simulink model "Scenario_3_v2"  (R2020b)
settings: Solver=ode1be  StartTime=0.0  StopTime=0.5  FixedStep=Ts  MaxStep=Ts/10  MinStep=Ts/40  RelTol=1e-3
values from neighbouring files (symbols this model uses):
  c0 = c0_zeb    (= 6.57988e-09)    [Scenario_17_parameters_v2.m]    (also in Scenario_1_parameters_v2.m; Scenario_2_parameters_v2.m; Scenario_3_parameters_v2.m)
  c0_hawk = 6.37282e-09    [Scenario_17_parameters_v2.m]    (also in Scenario_1_parameters_v2.m; Scenario_2_parameters_v2.m; Scenario_3_parameters_v2.m)
  c1 = c1_zeb    (= 9.15905e-09)    [Scenario_17_parameters_v2.m]    (also in Scenario_1_parameters_v2.m; Scenario_2_parameters_v2.m; Scenario_3_parameters_v2.m)
  c1_hawk = 8.76156e-09    [Scenario_17_parameters_v2.m]    (also in Scenario_1_parameters_v2.m; Scenario_2_parameters_v2.m; Scenario_3_parameters_v2.m)
  fg = 50    [Scenario_17_parameters_v2.m]    (also in Scenario_1_parameters_v2.m; Scenario_2_parameters_v2.m; Scenario_3_parameters_v2.m)
  G10gen = 0.90    (= 0.9)    [Scenario_3_parameters_v2.m]
  G12gen = 0.85    [Scenario_3_parameters_v2.m]
  G1gen = 0.4692    [Scenario_17_parameters_v2.m]    (also in Scenario_1_parameters_v2.m = 0.1; Scenario_2_parameters_v2.m = 0.298581; Scenario_3_parameters_v2.m = 0.65)
  G2gen = 0.80    (= 0.8)    [Scenario_1_parameters_v2.m]    (also in Scenario_2_parameters_v2.m = 0.7; Scenario_3_parameters_v2.m = 0.4)
  G3gen = 0.85    [Scenario_1_parameters_v2.m]    (also in Scenario_2_parameters_v2.m = 0.9; Scenario_3_parameters_v2.m = 0.6)
  G4gen = 0.65    [Scenario_3_parameters_v2.m]
  G5gen = 0.75    [Scenario_17_parameters_v2.m]    (also in Scenario_1_parameters_v2.m = 0.8; Scenario_2_parameters_v2.m = 0.8; Scenario_3_parameters_v2.m = 0.705)
  G6gen = 0.90    (= 0.9)    [Scenario_17_parameters_v2.m]    (also in Scenario_1_parameters_v2.m; Scenario_2_parameters_v2.m = 0.81797; Scenario_3_parameters_v2.m = 0.45)
  G7gen = 0.20    (= 0.2)    [Scenario_17_parameters_v2.m]    (also in Scenario_1_parameters_v2.m = 0.5227; Scenario_2_parameters_v2.m = 0.5098; Scenario_3_parameters_v2.m = 0.4)
  G8gen = 0.58    [Scenario_17_parameters_v2.m]    (also in Scenario_3_parameters_v2.m = 0.65)
  G9gen = 0.8833    [Scenario_17_parameters_v2.m]    (also in Scenario_3_parameters_v2.m = 0.9)
  Iovc = 1.2    [Scenario_17_parameters_v2.m]    (also in Scenario_1_parameters_v2.m; Scenario_2_parameters_v2.m; Scenario_3_parameters_v2.m)
  l0 = l0_zeb    (= 0.00368)    [Scenario_17_parameters_v2.m]    (also in Scenario_1_parameters_v2.m; Scenario_2_parameters_v2.m; Scenario_3_parameters_v2.m)
  l0_hawk = 0.00373    [Scenario_17_parameters_v2.m]    (also in Scenario_1_parameters_v2.m; Scenario_2_parameters_v2.m; Scenario_3_parameters_v2.m)
  l1 = l1_zeb    (= 0.00128)    [Scenario_17_parameters_v2.m]    (also in Scenario_1_parameters_v2.m; Scenario_2_parameters_v2.m; Scenario_3_parameters_v2.m)
  L10dem = 0.04    [Scenario_3_parameters_v2.m]
  L12dem = 0.01    [Scenario_17_parameters_v2.m]    (also in Scenario_3_parameters_v2.m = 0.02)
  L13dem = 0.01    [Scenario_3_parameters_v2.m]
  l1_hawk = 0.00133    [Scenario_17_parameters_v2.m]    (also in Scenario_1_parameters_v2.m; Scenario_2_parameters_v2.m; Scenario_3_parameters_v2.m)
  L1dem = 0.25    [Scenario_17_parameters_v2.m]    (also in Scenario_3_parameters_v2.m = 0.1)
  L3dem = 0.30    (= 0.3)    [Scenario_17_parameters_v2.m]    (also in Scenario_1_parameters_v2.m = 0.1; Scenario_2_parameters_v2.m = 0.1; Scenario_3_parameters_v2.m = 0.2)
  L5dem = 0.25    [Scenario_17_parameters_v2.m]    (also in Scenario_1_parameters_v2.m = 0.35; Scenario_2_parameters_v2.m = 0.35; Scenario_3_parameters_v2.m = 0.1)
  L6dem = 0.15    [Scenario_1_parameters_v2.m]    (also in Scenario_2_parameters_v2.m; Scenario_3_parameters_v2.m = 0.1)
  L7dem = 0.10    (= 0.1)    [Scenario_1_parameters_v2.m]    (also in Scenario_2_parameters_v2.m; Scenario_3_parameters_v2.m = 0.2)
  L9dem = 0.15    [Scenario_17_parameters_v2.m]    (also in Scenario_3_parameters_v2.m = 0.1)
  Pr = Sr*PF    (= 1600500000)    [Scenario_17_parameters_v2.m]    (also in Scenario_1_parameters_v2.m = 1472500000; Scenario_2_parameters_v2.m = 1805000000; Scenario_3_parameters_v2.m = 12740000000)
  Qr = sqrt(Sr^2 - Pr^2)    [Scenario_17_parameters_v2.m]    (also in Scenario_1_parameters_v2.m; Scenario_2_parameters_v2.m; Scenario_3_parameters_v2.m)
  r0 = r0_zeb    (= 0.39362)    [Scenario_17_parameters_v2.m]    (also in Scenario_1_parameters_v2.m; Scenario_2_parameters_v2.m; Scenario_3_parameters_v2.m)
  r0_hawk = 0.44587    [Scenario_17_parameters_v2.m]    (also in Scenario_1_parameters_v2.m; Scenario_2_parameters_v2.m; Scenario_3_parameters_v2.m)
  r1 = r1_zeb    (= 0.06862)    [Scenario_17_parameters_v2.m]    (also in Scenario_1_parameters_v2.m; Scenario_2_parameters_v2.m; Scenario_3_parameters_v2.m)
  r1_hawk = 0.12087    [Scenario_17_parameters_v2.m]    (also in Scenario_1_parameters_v2.m; Scenario_2_parameters_v2.m; Scenario_3_parameters_v2.m)
  Rtpu = Xtpu/40    (= 0.0025)    [Scenario_17_parameters_v2.m]    (also in Scenario_1_parameters_v2.m = 0.00375; Scenario_2_parameters_v2.m = 0.00375; Scenario_3_parameters_v2.m)
  S10non = 500e6    (= 500000000)    [Scenario_3_parameters_v2.m]
  S12non = 250e6    (= 250000000)    [Scenario_3_parameters_v2.m]
  S1non = 700e6    (= 700000000)    [Scenario_17_parameters_v2.m]    (also in Scenario_1_parameters_v2.m = 400000000; Scenario_2_parameters_v2.m = 400000000; Scenario_3_parameters_v2.m = 1000000000)
  S2non = 300e6    (= 300000000)    [Scenario_1_parameters_v2.m]    (also in Scenario_2_parameters_v2.m; Scenario_3_parameters_v2.m = 3000000000)
  S3non = 200e6    (= 200000000)    [Scenario_1_parameters_v2.m]    (also in Scenario_2_parameters_v2.m; Scenario_3_parameters_v2.m = 1000000000)
  S4non = 2000e6    (= 2000000000)    [Scenario_3_parameters_v2.m]
  S5non = 400e6    (= 400000000)    [Scenario_17_parameters_v2.m]    (also in Scenario_1_parameters_v2.m = 500000000; Scenario_2_parameters_v2.m = 500000000; Scenario_3_parameters_v2.m = 2000000000)
  S6non = 150e6    (= 150000000)    [Scenario_17_parameters_v2.m]    (also in Scenario_1_parameters_v2.m = 400000000; Scenario_2_parameters_v2.m = 400000000; Scenario_3_parameters_v2.m = 3000000000)
  S7non = 1500e6    (= 1500000000)    [Scenario_17_parameters_v2.m]    (also in Scenario_1_parameters_v2.m = 200000000; Scenario_2_parameters_v2.m = 200000000; Scenario_3_parameters_v2.m = 4000000000)
  S8non = 600e6    (= 600000000)    [Scenario_17_parameters_v2.m]    (also in Scenario_3_parameters_v2.m = 2000000000)
  S9non = 200e6    (= 200000000)    [Scenario_17_parameters_v2.m]    (also in Scenario_3_parameters_v2.m = 1500000000)
  tonvsc = 0    [Scenario_17_parameters_v2.m]    (also in Scenario_1_parameters_v2.m; Scenario_2_parameters_v2.m; Scenario_3_parameters_v2.m = 0.0001)
  Ts = 50e-6    (= 5e-05)    [Scenario_17_parameters_v2.m]    (also in Scenario_1_parameters_v2.m = 0.0002; Scenario_2_parameters_v2.m = 2e-05; Scenario_3_parameters_v2.m = 0.0001)
  Vhv = 220e3    (= 220000)    [Scenario_17_parameters_v2.m]    (also in Scenario_1_parameters_v2.m; Scenario_2_parameters_v2.m; Scenario_3_parameters_v2.m)
  Vmv = 22e3    (= 22000)    [Scenario_17_parameters_v2.m]    (also in Scenario_1_parameters_v2.m; Scenario_2_parameters_v2.m; Scenario_3_parameters_v2.m)
  w_pll = 2*pi*80    (= 502.654824574)    [Scenario_17_parameters_v2.m]    (also in Scenario_1_parameters_v2.m; Scenario_2_parameters_v2.m; Scenario_3_parameters_v2.m)
  wc1 = wsw1/10    (= 848.230016469)    [Scenario_17_parameters_v2.m]    (also in Scenario_1_parameters_v2.m; Scenario_2_parameters_v2.m; Scenario_3_parameters_v2.m)
  wdc1 = wc1/10    (= 84.8230016469)    [Scenario_17_parameters_v2.m]    (also in Scenario_1_parameters_v2.m; Scenario_2_parameters_v2.m; Scenario_3_parameters_v2.m)
  wpq1 = wc1/10    (= 84.8230016469)    [Scenario_17_parameters_v2.m]    (also in Scenario_1_parameters_v2.m; Scenario_2_parameters_v2.m; Scenario_3_parameters_v2.m)
  wsw1 = ksw1*2*pi*fg    (= 8482.30016469)    [Scenario_17_parameters_v2.m]    (also in Scenario_1_parameters_v2.m; Scenario_2_parameters_v2.m; Scenario_3_parameters_v2.m)
  Xtpu = 0.10    (= 0.1)    [Scenario_17_parameters_v2.m]    (also in Scenario_1_parameters_v2.m = 0.15; Scenario_2_parameters_v2.m = 0.15; Scenario_3_parameters_v2.m)
undefined symbols (not defined in the file or in its folder): D11, Delta
libraries: powerlib x428, simulink_extras x272, powerlib_meascontrol x194, pid_lib x105, simulink x60, eeTransforms x54, spsFirstOrderFilterLib x36, eePwmGeneratorTwoLevel x9
(part 10 of 40)

== system Scenario_3_v2/G7/VSC v2/VSC Model ==
  Ref : Inport
  EMT AVG : Subsystem  VariantControl=EMT_AVG
      settings: PortSchema="{\"entries\":[{\"content\":{\"sides\":[{\"content\":{\"connectorIds\":[\"LConn1\",\"LConn2\",\"LConn3\"]},\"type\":\"ConnectorPlacement.EquallySpacedRectSide\",\"uuid\":\"96043b84-a665-4cb2-a938-d6633d7ee474\"},{\"content\":{\"connectorIds\":[\"In1\"],\"side\":\"RIGHT\"},\"type\":\"ConnectorPlacement.EquallySpacedRectSide\",\"uuid\":\"064d463f-c23a-42ac-89ce-8dea3d446214\"},{\"content\":{\"connectorIds\":[],\"side\":\"TOP\"},\"type\":\"ConnectorPlacement.EquallySpacedRectSide\",\"uuid\":\"95ef669c-c6ed-44c3-8b69-447906728b6d\"}]},\"type\":\"ConnectorPlacement.EquallySpacedConnector\",\"uuid\":\"ea66db09-64d7-4d7e-ba7b-d769c56e2dbd\"}],\"packageUris\":[\"http://schema.mathworks.com/mf0/Connector/19700101\"],\"version\":\"1.0\"}"
  EMT SW : Subsystem  VariantControl=EMT_SW
      settings: PortSchema="{\"entries\":[{\"content\":{\"sides\":[{\"content\":{\"connectorIds\":[\"LConn1\",\"LConn2\",\"LConn3\"]},\"type\":\"ConnectorPlacement.EquallySpacedRectSide\",\"uuid\":\"96043b84-a665-4cb2-a938-d6633d7ee474\"},{\"content\":{\"connectorIds\":[\"In1\"],\"side\":\"RIGHT\"},\"type\":\"ConnectorPlacement.EquallySpacedRectSide\",\"uuid\":\"064d463f-c23a-42ac-89ce-8dea3d446214\"},{\"content\":{\"connectorIds\":[],\"side\":\"TOP\"},\"type\":\"ConnectorPlacement.EquallySpacedRectSide\",\"uuid\":\"95ef669c-c6ed-44c3-8b69-447906728b6d\"}]},\"type\":\"ConnectorPlacement.EquallySpacedConnector\",\"uuid\":\"ea66db09-64d7-4d7e-ba7b-d769c56e2dbd\"}],\"packageUris\":[\"http://schema.mathworks.com/mf0/Connector/19700101\"],\"version\":\"1.0\"}"
  Phasor : Subsystem  VariantControl=Phasor
      settings: PortSchema="{\"entries\":[{\"content\":{\"sides\":[{\"content\":{\"connectorIds\":[\"LConn1\",\"LConn2\",\"LConn3\"]},\"type\":\"ConnectorPlacement.EquallySpacedRectSide\",\"uuid\":\"96043b84-a665-4cb2-a938-d6633d7ee474\"},{\"content\":{\"connectorIds\":[\"In1\"],\"side\":\"RIGHT\"},\"type\":\"ConnectorPlacement.EquallySpacedRectSide\",\"uuid\":\"064d463f-c23a-42ac-89ce-8dea3d446214\"},{\"content\":{\"connectorIds\":[],\"side\":\"TOP\"},\"type\":\"ConnectorPlacement.EquallySpacedRectSide\",\"uuid\":\"95ef669c-c6ed-44c3-8b69-447906728b6d\"}]},\"type\":\"ConnectorPlacement.EquallySpacedConnector\",\"uuid\":\"ea66db09-64d7-4d7e-ba7b-d769c56e2dbd\"}],\"packageUris\":[\"http://schema.mathworks.com/mf0/Connector/19700101\"],\"version\":\"1.0\"}"
  A : PMIOPort  Side=Left
  B : PMIOPort  Port=2  Side=Left
  C : PMIOPort  Port=3  Side=Left

== system Scenario_3_v2/G7/VSC v2/output signals ==
  Vs : Inport
  Is : Inport  Port=2
  control : Inport  Port=3
  Bus Creator : BusCreator  Inputs=15
  Demux : Demux  Outputs=13
  m : Outport
  wires:
  Bus Creator/1 -> m/1
  control/1 -> Demux/1
  Vs/1 -> Bus Creator/1  "Vabc"
  Is/1 -> Bus Creator/2  "Iabc"
  Demux/1 -> Bus Creator/3  "vqp"
  Demux/2 -> Bus Creator/4  "vdp"
  Demux/3 -> Bus Creator/5  "vqn"
  Demux/4 -> Bus Creator/6  "vdn"
  Demux/5 -> Bus Creator/7  "iqp"
  Demux/6 -> Bus Creator/8  "idp"
  Demux/7 -> Bus Creator/9  "iqn"
  Demux/8 -> Bus Creator/10  "idn"
  Demux/9 -> Bus Creator/11  "f"
  Demux/10 -> Bus Creator/12  "Pdq"
  Demux/11 -> Bus Creator/13  "Qdq"
  Demux/12 -> Bus Creator/14  "Pabc"
  Demux/13 -> Bus Creator/15  "Qabc"

== system Scenario_3_v2/G9/VSC v2/VI measurement ==
  Current Measurement : powerlib/Measurements/Current Measurement  PhasorSimulation=off  OutputType=Complex  PSBequivalent=0
  Current Measurement1 : powerlib/Measurements/Current Measurement  PhasorSimulation=off  OutputType=Complex  PSBequivalent=0
  Current Measurement2 : powerlib/Measurements/Current Measurement  PhasorSimulation=off  OutputType=Complex  PSBequivalent=0
  Ground : powerlib/Elements/Ground  LConnTagsString=a
  Ground1 : powerlib/Elements/Ground  LConnTagsString=a
  Ground2 : powerlib/Elements/Ground  LConnTagsString=a
  Mux : Mux  Inputs=3
  Mux1 : Mux  Inputs=3
  Voltage Measurement : powerlib/Measurements/Voltage Measurement  PhasorSimulation=off  OutputType=Complex  PSBequivalent=0
  Voltage Measurement1 : powerlib/Measurements/Voltage Measurement  PhasorSimulation=off  OutputType=Complex  PSBequivalent=0
  Voltage Measurement2 : powerlib/Measurements/Voltage Measurement  PhasorSimulation=off  OutputType=Complex  PSBequivalent=0
  A : PMIOPort  Side=Left
  B : PMIOPort  Port=2  Side=Left
  C : PMIOPort  Port=3  Side=Left
  a : PMIOPort  Port=4  Side=Right
  b : PMIOPort  Port=5  Side=Right
  c : PMIOPort  Port=6  Side=Right
  Vs : Outport
  Is : Outport  Port=2
  wires:
  Mux1/1 -> Is/1
  Mux/1 -> Vs/1
  Voltage Measurement1/1 -> Mux/2
  Voltage Measurement2/1 -> Mux/3
  Current Measurement2/1 -> Mux1/3
  Voltage Measurement/1 -> Mux/1
  Current Measurement/1 -> Mux1/1
  Current Measurement1/1 -> Mux1/2
  connections:
  Voltage Measurement/LConn1 -- Current Measurement/LConn1 -- A/RConn1
  Current Measurement2/LConn1 -- Voltage Measurement2/LConn1 -- C/RConn1
  Current Measurement1/LConn1 -- Voltage Measurement1/LConn1 -- B/RConn1
  Current Measurement1/RConn1 -- b/RConn1
  Current Measurement/RConn1 -- a/RConn1
  Ground/LConn1 -- Voltage Measurement/LConn2
  Current Measurement2/RConn1 -- c/RConn1
  Ground1/LConn1 -- Voltage Measurement1/LConn2
  Ground2/LConn1 -- Voltage Measurement2/LConn2

== system Scenario_3_v2/G9/VSC v2/VSC Control ==
  Block : Inport
  Vabc : Inport  Port=2
  Iabc : Inport  Port=3
  Pset : Inport  Port=4
  Qset : Inport  Port=5
  Edc : Inport  Port=6
  Control loops : Subsystem  Variant=on  VariantControlMode=label  LabelModeActiveChoice=EMT_and_QEMT
  Measurements : Subsystem  Variant=on  VariantControlMode=label  LabelModeActiveChoice=EMT
  Modulation : Subsystem  Variant=on  VariantControlMode=label  LabelModeActiveChoice=EMT_AVG
  Mux : Mux  Inputs=2
  Ref : Outport
  m : Outport  Port=2
  wires:
  Control loops/2(iqd+-ref) -> Modulation/3(iqd+-*)
  Control loops/1(vqd+-ref) -> Modulation/2(vqd+-*)
  [PQabc] -> Mux/2
  Measurements/5(PQabc) -> [PQabc]
  Modulation/1(Ref) -> Ref/1
  Measurements/4(theta) -> [theta]
  Vabc/1 -> Measurements/1(Vabc)
  Measurements/1(vqd+-) -> Control loops/3(vqd+-), [vqdpn]
  Measurements/2(iqd+-) -> Control loops/4(iqd+-)
  Measurements/3(freq) -> Control loops/5(freq)
  [theta] -> Modulation/4(theta)
  [vqdpn] -> Modulation/1(vqd+-)
  Iabc/1 -> Measurements/2(Iabc)
  Mux/1 -> m/1
  Control loops/3(m) -> Mux/1
  Pset/1 -> Control loops/1(Pset)
  Qset/1 -> Control loops/2(Qset)
  Block/1 -> Control loops/6(Block)
  Edc/1 -> Control loops/7(Edc)

== system Scenario_3_v2/G9/VSC v2/VSC Model ==
  Ref : Inport
  EMT AVG : Subsystem  VariantControl=EMT_AVG
      settings: PortSchema="{\"entries\":[{\"content\":{\"sides\":[{\"content\":{\"connectorIds\":[\"LConn1\",\"LConn2\",\"LConn3\"]},\"type\":\"ConnectorPlacement.EquallySpacedRectSide\",\"uuid\":\"96043b84-a665-4cb2-a938-d6633d7ee474\"},{\"content\":{\"connectorIds\":[\"In1\"],\"side\":\"RIGHT\"},\"type\":\"ConnectorPlacement.EquallySpacedRectSide\",\"uuid\":\"064d463f-c23a-42ac-89ce-8dea3d446214\"},{\"content\":{\"connectorIds\":[],\"side\":\"TOP\"},\"type\":\"ConnectorPlacement.EquallySpacedRectSide\",\"uuid\":\"95ef669c-c6ed-44c3-8b69-447906728b6d\"}]},\"type\":\"ConnectorPlacement.EquallySpacedConnector\",\"uuid\":\"ea66db09-64d7-4d7e-ba7b-d769c56e2dbd\"}],\"packageUris\":[\"http://schema.mathworks.com/mf0/Connector/19700101\"],\"version\":\"1.0\"}"
  EMT SW : Subsystem  VariantControl=EMT_SW
      settings: PortSchema="{\"entries\":[{\"content\":{\"sides\":[{\"content\":{\"connectorIds\":[\"LConn1\",\"LConn2\",\"LConn3\"]},\"type\":\"ConnectorPlacement.EquallySpacedRectSide\",\"uuid\":\"96043b84-a665-4cb2-a938-d6633d7ee474\"},{\"content\":{\"connectorIds\":[\"In1\"],\"side\":\"RIGHT\"},\"type\":\"ConnectorPlacement.EquallySpacedRectSide\",\"uuid\":\"064d463f-c23a-42ac-89ce-8dea3d446214\"},{\"content\":{\"connectorIds\":[],\"side\":\"TOP\"},\"type\":\"ConnectorPlacement.EquallySpacedRectSide\",\"uuid\":\"95ef669c-c6ed-44c3-8b69-447906728b6d\"}]},\"type\":\"ConnectorPlacement.EquallySpacedConnector\",\"uuid\":\"ea66db09-64d7-4d7e-ba7b-d769c56e2dbd\"}],\"packageUris\":[\"http://schema.mathworks.com/mf0/Connector/19700101\"],\"version\":\"1.0\"}"
  Phasor : Subsystem  VariantControl=Phasor
      settings: PortSchema="{\"entries\":[{\"content\":{\"sides\":[{\"content\":{\"connectorIds\":[\"LConn1\",\"LConn2\",\"LConn3\"]},\"type\":\"ConnectorPlacement.EquallySpacedRectSide\",\"uuid\":\"96043b84-a665-4cb2-a938-d6633d7ee474\"},{\"content\":{\"connectorIds\":[\"In1\"],\"side\":\"RIGHT\"},\"type\":\"ConnectorPlacement.EquallySpacedRectSide\",\"uuid\":\"064d463f-c23a-42ac-89ce-8dea3d446214\"},{\"content\":{\"connectorIds\":[],\"side\":\"TOP\"},\"type\":\"ConnectorPlacement.EquallySpacedRectSide\",\"uuid\":\"95ef669c-c6ed-44c3-8b69-447906728b6d\"}]},\"type\":\"ConnectorPlacement.EquallySpacedConnector\",\"uuid\":\"ea66db09-64d7-4d7e-ba7b-d769c56e2dbd\"}],\"packageUris\":[\"http://schema.mathworks.com/mf0/Connector/19700101\"],\"version\":\"1.0\"}"
  A : PMIOPort  Side=Left
  B : PMIOPort  Port=2  Side=Left
  C : PMIOPort  Port=3  Side=Left

== system Scenario_3_v2/G9/VSC v2/output signals ==
  Vs : Inport
  Is : Inport  Port=2
  control : Inport  Port=3
  Bus Creator : BusCreator  Inputs=15
  Demux : Demux  Outputs=13
  m : Outport
  wires:
  Bus Creator/1 -> m/1
  control/1 -> Demux/1
  Vs/1 -> Bus Creator/1  "Vabc"
  Is/1 -> Bus Creator/2  "Iabc"
  Demux/1 -> Bus Creator/3  "vqp"
  Demux/2 -> Bus Creator/4  "vdp"
  Demux/3 -> Bus Creator/5  "vqn"
  Demux/4 -> Bus Creator/6  "vdn"
  Demux/5 -> Bus Creator/7  "iqp"
  Demux/6 -> Bus Creator/8  "idp"
  Demux/7 -> Bus Creator/9  "iqn"
  Demux/8 -> Bus Creator/10  "idn"
  Demux/9 -> Bus Creator/11  "f"
  Demux/10 -> Bus Creator/12  "Pdq"
  Demux/11 -> Bus Creator/13  "Qdq"
  Demux/12 -> Bus Creator/14  "Pabc"
  Demux/13 -> Bus Creator/15  "Qabc"

== system Scenario_3_v2/HVDC/VSC1 v2/VI measurement ==
  Current Measurement : powerlib/Measurements/Current Measurement  PhasorSimulation=off  OutputType=Complex  PSBequivalent=0
  Current Measurement1 : powerlib/Measurements/Current Measurement  PhasorSimulation=off  OutputType=Complex  PSBequivalent=0
  Current Measurement2 : powerlib/Measurements/Current Measurement  PhasorSimulation=off  OutputType=Complex  PSBequivalent=0
  Ground : powerlib/Elements/Ground  LConnTagsString=a
  Ground1 : powerlib/Elements/Ground  LConnTagsString=a
  Ground2 : powerlib/Elements/Ground  LConnTagsString=a
  Mux : Mux  Inputs=3
  Mux1 : Mux  Inputs=3
  Voltage Measurement : powerlib/Measurements/Voltage Measurement  PhasorSimulation=off  OutputType=Complex  PSBequivalent=0
  Voltage Measurement1 : powerlib/Measurements/Voltage Measurement  PhasorSimulation=off  OutputType=Complex  PSBequivalent=0
  Voltage Measurement2 : powerlib/Measurements/Voltage Measurement  PhasorSimulation=off  OutputType=Complex  PSBequivalent=0
  A : PMIOPort  Side=Left
  B : PMIOPort  Port=2  Side=Left
  C : PMIOPort  Port=3  Side=Left
  a : PMIOPort  Port=4  Side=Right
  b : PMIOPort  Port=5  Side=Right
  c : PMIOPort  Port=6  Side=Right
  Vs : Outport
  Is : Outport  Port=2
  wires:
  Mux1/1 -> Is/1
  Mux/1 -> Vs/1
  Voltage Measurement1/1 -> Mux/2
  Voltage Measurement2/1 -> Mux/3
  Current Measurement2/1 -> Mux1/3
  Voltage Measurement/1 -> Mux/1
  Current Measurement/1 -> Mux1/1
  Current Measurement1/1 -> Mux1/2
  connections:
  Voltage Measurement/LConn1 -- Current Measurement/LConn1 -- A/RConn1
  Current Measurement2/LConn1 -- Voltage Measurement2/LConn1 -- C/RConn1
  Current Measurement1/LConn1 -- Voltage Measurement1/LConn1 -- B/RConn1
  Current Measurement1/RConn1 -- b/RConn1
  Current Measurement/RConn1 -- a/RConn1
  Ground/LConn1 -- Voltage Measurement/LConn2
  Current Measurement2/RConn1 -- c/RConn1
  Ground1/LConn1 -- Voltage Measurement1/LConn2
  Ground2/LConn1 -- Voltage Measurement2/LConn2

== system Scenario_3_v2/HVDC/VSC1 v2/VSC Control ==
  Block : Inport
  Vabc : Inport  Port=2
  Iabc : Inport  Port=3
  Pset : Inport  Port=4
  Qset : Inport  Port=5
  Control loops : Subsystem  Variant=on  VariantControlMode=label  LabelModeActiveChoice=EMT_and_QEMT
  Measurements : Subsystem  Variant=on  VariantControlMode=label  LabelModeActiveChoice=EMT
  Modulation : Subsystem  Variant=on  VariantControlMode=label  LabelModeActiveChoice=EMT_AVG
  Mux : Mux  Inputs=2
  Ref : Outport
  m : Outport  Port=2
  wires:
  Control loops/2(iqd+-ref) -> Modulation/3(iqd+-*)
  Control loops/1(vqd+-ref) -> Modulation/2(vqd+-*)
  [PQabc] -> Mux/2
  Measurements/5(PQabc) -> [PQabc]
  Modulation/1(Ref) -> Ref/1
  Measurements/4(theta) -> [theta]
  Vabc/1 -> Measurements/1(Vabc)
  Measurements/1(vqd+-) -> Control loops/3(vqd+-), [vqdpn]
  Measurements/2(iqd+-) -> Control loops/4(iqd+-)
  Measurements/3(freq) -> Control loops/5(freq)
  [theta] -> Modulation/4(theta)
  [vqdpn] -> Modulation/1(vqd+-)
  Iabc/1 -> Measurements/2(Iabc)
  Mux/1 -> m/1
  Control loops/3(m) -> Mux/1
  Pset/1 -> Control loops/1(Pset)
  Qset/1 -> Control loops/2(Qset)
  Block/1 -> Control loops/6(Block)

== system Scenario_3_v2/HVDC/VSC1 v2/VSC Model ==
  Ref : Inport
  EMT AVG : Subsystem  VariantControl=EMT_AVG
      settings: PortSchema="{\"entries\":[{\"content\":{\"sides\":[{\"content\":{\"connectorIds\":[\"LConn1\",\"LConn2\",\"LConn3\"]},\"type\":\"ConnectorPlacement.EquallySpacedRectSide\",\"uuid\":\"96043b84-a665-4cb2-a938-d6633d7ee474\"},{\"content\":{\"connectorIds\":[\"In1\"],\"side\":\"RIGHT\"},\"type\":\"ConnectorPlacement.EquallySpacedRectSide\",\"uuid\":\"064d463f-c23a-42ac-89ce-8dea3d446214\"},{\"content\":{\"connectorIds\":[],\"side\":\"TOP\"},\"type\":\"ConnectorPlacement.EquallySpacedRectSide\",\"uuid\":\"95ef669c-c6ed-44c3-8b69-447906728b6d\"}]},\"type\":\"ConnectorPlacement.EquallySpacedConnector\",\"uuid\":\"ea66db09-64d7-4d7e-ba7b-d769c56e2dbd\"}],\"packageUris\":[\"http://schema.mathworks.com/mf0/Connector/19700101\"],\"version\":\"1.0\"}"
  EMT SW : Subsystem  VariantControl=EMT_SW
      settings: PortSchema="{\"entries\":[{\"content\":{\"sides\":[{\"content\":{\"connectorIds\":[\"LConn1\",\"LConn2\",\"LConn3\"]},\"type\":\"ConnectorPlacement.EquallySpacedRectSide\",\"uuid\":\"96043b84-a665-4cb2-a938-d6633d7ee474\"},{\"content\":{\"connectorIds\":[\"In1\"],\"side\":\"RIGHT\"},\"type\":\"ConnectorPlacement.EquallySpacedRectSide\",\"uuid\":\"064d463f-c23a-42ac-89ce-8dea3d446214\"},{\"content\":{\"connectorIds\":[],\"side\":\"TOP\"},\"type\":\"ConnectorPlacement.EquallySpacedRectSide\",\"uuid\":\"95ef669c-c6ed-44c3-8b69-447906728b6d\"}]},\"type\":\"ConnectorPlacement.EquallySpacedConnector\",\"uuid\":\"ea66db09-64d7-4d7e-ba7b-d769c56e2dbd\"}],\"packageUris\":[\"http://schema.mathworks.com/mf0/Connector/19700101\"],\"version\":\"1.0\"}"
  Phasor : Subsystem  VariantControl=Phasor
      settings: PortSchema="{\"entries\":[{\"content\":{\"sides\":[{\"content\":{\"connectorIds\":[\"LConn1\",\"LConn2\",\"LConn3\"]},\"type\":\"ConnectorPlacement.EquallySpacedRectSide\",\"uuid\":\"96043b84-a665-4cb2-a938-d6633d7ee474\"},{\"content\":{\"connectorIds\":[\"In1\"],\"side\":\"RIGHT\"},\"type\":\"ConnectorPlacement.EquallySpacedRectSide\",\"uuid\":\"064d463f-c23a-42ac-89ce-8dea3d446214\"},{\"content\":{\"connectorIds\":[],\"side\":\"TOP\"},\"type\":\"ConnectorPlacement.EquallySpacedRectSide\",\"uuid\":\"95ef669c-c6ed-44c3-8b69-447906728b6d\"}]},\"type\":\"ConnectorPlacement.EquallySpacedConnector\",\"uuid\":\"ea66db09-64d7-4d7e-ba7b-d769c56e2dbd\"}],\"packageUris\":[\"http://schema.mathworks.com/mf0/Connector/19700101\"],\"version\":\"1.0\"}"
  A : PMIOPort  Side=Left
  B : PMIOPort  Port=2  Side=Left
  C : PMIOPort  Port=3  Side=Left

== system Scenario_3_v2/HVDC/VSC1 v2/output signals ==
  Vs : Inport
  Is : Inport  Port=2
  control : Inport  Port=3
  Bus Creator : BusCreator  Inputs=15
  Demux : Demux  Outputs=13
  m : Outport
  wires:
  Bus Creator/1 -> m/1
  control/1 -> Demux/1
  Vs/1 -> Bus Creator/1  "Vabc"
  Is/1 -> Bus Creator/2  "Iabc"
  Demux/1 -> Bus Creator/3  "vqp"
  Demux/2 -> Bus Creator/4  "vdp"
  Demux/3 -> Bus Creator/5  "vqn"
  Demux/4 -> Bus Creator/6  "vdn"
  Demux/5 -> Bus Creator/7  "iqp"
  Demux/6 -> Bus Creator/8  "idp"
  Demux/7 -> Bus Creator/9  "iqn"
  Demux/8 -> Bus Creator/10  "idn"
  Demux/9 -> Bus Creator/11  "f"
  Demux/10 -> Bus Creator/12  "Pdq"
  Demux/11 -> Bus Creator/13  "Qdq"
  Demux/12 -> Bus Creator/14  "Pabc"
  Demux/13 -> Bus Creator/15  "Qabc"

== system Scenario_3_v2/HVDC/VSC2 v2/VI measurement ==
  Current Measurement : powerlib/Measurements/Current Measurement  PhasorSimulation=off  OutputType=Complex  PSBequivalent=0
  Current Measurement1 : powerlib/Measurements/Current Measurement  PhasorSimulation=off  OutputType=Complex  PSBequivalent=0
  Current Measurement2 : powerlib/Measurements/Current Measurement  PhasorSimulation=off  OutputType=Complex  PSBequivalent=0
  Ground : powerlib/Elements/Ground  LConnTagsString=a
  Ground1 : powerlib/Elements/Ground  LConnTagsString=a
  Ground2 : powerlib/Elements/Ground  LConnTagsString=a
  Mux : Mux  Inputs=3
  Mux1 : Mux  Inputs=3
  Voltage Measurement : powerlib/Measurements/Voltage Measurement  PhasorSimulation=off  OutputType=Complex  PSBequivalent=0
  Voltage Measurement1 : powerlib/Measurements/Voltage Measurement  PhasorSimulation=off  OutputType=Complex  PSBequivalent=0
  Voltage Measurement2 : powerlib/Measurements/Voltage Measurement  PhasorSimulation=off  OutputType=Complex  PSBequivalent=0
  A : PMIOPort  Side=Left
  B : PMIOPort  Port=2  Side=Left
  C : PMIOPort  Port=3  Side=Left
  a : PMIOPort  Port=4  Side=Right
  b : PMIOPort  Port=5  Side=Right
  c : PMIOPort  Port=6  Side=Right
  Vs : Outport
  Is : Outport  Port=2
  wires:
  Mux1/1 -> Is/1
  Mux/1 -> Vs/1
  Voltage Measurement1/1 -> Mux/2
  Voltage Measurement2/1 -> Mux/3
  Current Measurement2/1 -> Mux1/3
  Voltage Measurement/1 -> Mux/1
  Current Measurement/1 -> Mux1/1
  Current Measurement1/1 -> Mux1/2
  connections:
  Voltage Measurement/LConn1 -- Current Measurement/LConn1 -- A/RConn1
  Current Measurement2/LConn1 -- Voltage Measurement2/LConn1 -- C/RConn1
  Current Measurement1/LConn1 -- Voltage Measurement1/LConn1 -- B/RConn1
  Current Measurement1/RConn1 -- b/RConn1
  Current Measurement/RConn1 -- a/RConn1
  Ground/LConn1 -- Voltage Measurement/LConn2
  Current Measurement2/RConn1 -- c/RConn1
  Ground1/LConn1 -- Voltage Measurement1/LConn2
  Ground2/LConn1 -- Voltage Measurement2/LConn2

== system Scenario_3_v2/HVDC/VSC2 v2/VSC Control ==
  Block : Inport
  Vabc : Inport  Port=2
  Iabc : Inport  Port=3
  Pset : Inport  Port=4
  Qset : Inport  Port=5
  Edc : Inport  Port=6
  Control loops : Subsystem  Variant=on  VariantControlMode=label  LabelModeActiveChoice=EMT_and_QEMT
  Measurements : Subsystem  Variant=on  VariantControlMode=label  LabelModeActiveChoice=EMT
  Modulation : Subsystem  Variant=on  VariantControlMode=label  LabelModeActiveChoice=EMT_AVG
  Mux : Mux  Inputs=2
  Ref : Outport
  m : Outport  Port=2
  wires:
  Control loops/2(iqd+-ref) -> Modulation/3(iqd+-*)
  Control loops/1(vqd+-ref) -> Modulation/2(vqd+-*)
  [PQabc] -> Mux/2
  Measurements/5(PQabc) -> [PQabc]
  Modulation/1(Ref) -> Ref/1
  Measurements/4(theta) -> [theta]
  Vabc/1 -> Measurements/1(Vabc)
  Measurements/1(vqd+-) -> Control loops/3(vqd+-), [vqdpn]
  Measurements/2(iqd+-) -> Control loops/4(iqd+-)
  Measurements/3(freq) -> Control loops/5(freq)
  [theta] -> Modulation/4(theta)
  [vqdpn] -> Modulation/1(vqd+-)
  Iabc/1 -> Measurements/2(Iabc)
  Mux/1 -> m/1
  Control loops/3(m) -> Mux/1
  Pset/1 -> Control loops/1(Pset)
  Qset/1 -> Control loops/2(Qset)
  Block/1 -> Control loops/6(Block)
  Edc/1 -> Control loops/7(Edc)

== system Scenario_3_v2/HVDC/VSC2 v2/VSC Model ==
  Ref : Inport
  EMT AVG : Subsystem  VariantControl=EMT_AVG
      settings: PortSchema="{\"entries\":[{\"content\":{\"sides\":[{\"content\":{\"connectorIds\":[\"LConn1\",\"LConn2\",\"LConn3\"]},\"type\":\"ConnectorPlacement.EquallySpacedRectSide\",\"uuid\":\"96043b84-a665-4cb2-a938-d6633d7ee474\"},{\"content\":{\"connectorIds\":[\"In1\"],\"side\":\"RIGHT\"},\"type\":\"ConnectorPlacement.EquallySpacedRectSide\",\"uuid\":\"064d463f-c23a-42ac-89ce-8dea3d446214\"},{\"content\":{\"connectorIds\":[],\"side\":\"TOP\"},\"type\":\"ConnectorPlacement.EquallySpacedRectSide\",\"uuid\":\"95ef669c-c6ed-44c3-8b69-447906728b6d\"}]},\"type\":\"ConnectorPlacement.EquallySpacedConnector\",\"uuid\":\"ea66db09-64d7-4d7e-ba7b-d769c56e2dbd\"}],\"packageUris\":[\"http://schema.mathworks.com/mf0/Connector/19700101\"],\"version\":\"1.0\"}"
  EMT SW : Subsystem  VariantControl=EMT_SW
      settings: PortSchema="{\"entries\":[{\"content\":{\"sides\":[{\"content\":{\"connectorIds\":[\"LConn1\",\"LConn2\",\"LConn3\"]},\"type\":\"ConnectorPlacement.EquallySpacedRectSide\",\"uuid\":\"96043b84-a665-4cb2-a938-d6633d7ee474\"},{\"content\":{\"connectorIds\":[\"In1\"],\"side\":\"RIGHT\"},\"type\":\"ConnectorPlacement.EquallySpacedRectSide\",\"uuid\":\"064d463f-c23a-42ac-89ce-8dea3d446214\"},{\"content\":{\"connectorIds\":[],\"side\":\"TOP\"},\"type\":\"ConnectorPlacement.EquallySpacedRectSide\",\"uuid\":\"95ef669c-c6ed-44c3-8b69-447906728b6d\"}]},\"type\":\"ConnectorPlacement.EquallySpacedConnector\",\"uuid\":\"ea66db09-64d7-4d7e-ba7b-d769c56e2dbd\"}],\"packageUris\":[\"http://schema.mathworks.com/mf0/Connector/19700101\"],\"version\":\"1.0\"}"
  Phasor : Subsystem  VariantControl=Phasor
      settings: PortSchema="{\"entries\":[{\"content\":{\"sides\":[{\"content\":{\"connectorIds\":[\"LConn1\",\"LConn2\",\"LConn3\"]},\"type\":\"ConnectorPlacement.EquallySpacedRectSide\",\"uuid\":\"96043b84-a665-4cb2-a938-d6633d7ee474\"},{\"content\":{\"connectorIds\":[\"In1\"],\"side\":\"RIGHT\"},\"type\":\"ConnectorPlacement.EquallySpacedRectSide\",\"uuid\":\"064d463f-c23a-42ac-89ce-8dea3d446214\"},{\"content\":{\"connectorIds\":[],\"side\":\"TOP\"},\"type\":\"ConnectorPlacement.EquallySpacedRectSide\",\"uuid\":\"95ef669c-c6ed-44c3-8b69-447906728b6d\"}]},\"type\":\"ConnectorPlacement.EquallySpacedConnector\",\"uuid\":\"ea66db09-64d7-4d7e-ba7b-d769c56e2dbd\"}],\"packageUris\":[\"http://schema.mathworks.com/mf0/Connector/19700101\"],\"version\":\"1.0\"}"
  A : PMIOPort  Side=Left
  B : PMIOPort  Port=2  Side=Left
  C : PMIOPort  Port=3  Side=Left

== system Scenario_3_v2/HVDC/VSC2 v2/output signals ==
  Vs : Inport
  Is : Inport  Port=2
  control : Inport  Port=3
  Bus Creator : BusCreator  Inputs=15
  Demux : Demux  Outputs=13
  m : Outport
  wires:
  Bus Creator/1 -> m/1
  control/1 -> Demux/1
  Vs/1 -> Bus Creator/1  "Vabc"
  Is/1 -> Bus Creator/2  "Iabc"
  Demux/1 -> Bus Creator/3  "vqp"
  Demux/2 -> Bus Creator/4  "vdp"
  Demux/3 -> Bus Creator/5  "vqn"
  Demux/4 -> Bus Creator/6  "vdn"
  Demux/5 -> Bus Creator/7  "iqp"
  Demux/6 -> Bus Creator/8  "idp"
  Demux/7 -> Bus Creator/9  "iqn"
  Demux/8 -> Bus Creator/10  "idn"
  Demux/9 -> Bus Creator/11  "f"
  Demux/10 -> Bus Creator/12  "Pdq"
  Demux/11 -> Bus Creator/13  "Qdq"
  Demux/12 -> Bus Creator/14  "Pabc"
  Demux/13 -> Bus Creator/15  "Qabc"

== system Scenario_3_v2/AC network/Exciter System/SEXS/1st ord transfer fcn windup limiter ==
  note: First order transfer function with windup limiter (non-saturated output)
  In1 : Inport
  Compare To Constant : simulink/Logic and Bit Operations/Compare To Constant  relop=<=  const=Vmax  OutDataTypeStr=boolean
  Compare To Constant1 : simulink/Logic and Bit Operations/Compare To Constant  relop=>=  const=Vmin  OutDataTypeStr=boolean
  OR : Logic  Operator=OR  IconShape=distinctive  AllPortsSameDT=off  OutDataTypeStr=boolean
  Sample and Hold1 : powerlib_meascontrol/Additional Components/Sample and Hold  ic=0  Ts=0
      settings: SourceProductBaseCode=PS
  Saturation1 : Saturate  UpperLimit=Vmax  LowerLimit=Vmin
  Transfer Fcn (with initial outputs)2 : simulink_extras/Additional Linear/Transfer Fcn (with initial outputs)  N=[Gain]  D=[tau 1]  Y0=y0  U0=y0/Gain
  Out1 : Outport
  wires:
  Sample and Hold1/1 -> Transfer Fcn (with initial outputs)2/1
  Transfer Fcn (with initial outputs)2/1 -> Saturation1/1, Compare To Constant1/1, Compare To Constant/1
  In1/1 -> Sample and Hold1/1
  Compare To Constant/1 -> OR/1
  Compare To Constant1/1 -> OR/2
  OR/1 -> Sample and Hold1/2
  Saturation1/1 -> Out1/1

== system Scenario_3_v2/G1/VSC v2/VSC Control/Control loops ==
  note: 1) Add Subsystem or Model blocks as valid variant choices.
      | 2) You cannot connect blocks at this level. At simulation, connectivity is automatically
      | determined, based on the active variant and port name matching.
  Pset : Inport
  Qset : Inport  Port=2
  vqd+- : Inport  Port=3
  iqd+- : Inport  Port=4
  freq : Inport  Port=5
  Block : Inport  Port=6
  Edc : Inport  Port=7
  Phasor I 1st : Subsystem  VariantControl=Phasor_I_1st
  Phasor I ref : Subsystem  VariantControl=Phasor_I_ref
  Phasor PQ 1st : Subsystem  VariantControl=Phasor_PQ
  "SW, EMT AVG, Phasor Quasi-EMT" : Subsystem  VariantControl=EMT_and_QEMT
  vqd+-ref : Outport
  iqd+-ref : Outport  Port=2
  m : Outport  Port=3

== system Scenario_3_v2/G1/VSC v2/VSC Control/Measurements ==
  note: 1) Add Subsystem or Model blocks as valid variant choices.
      | 2) You cannot connect blocks at this level. At simulation, connectivity is automatically
      | determined, based on the active variant and port name matching.
  Vabc : Inport
  Iabc : Inport  Port=2
  EMT : Subsystem  VariantControl=EMT
  Phasor : Subsystem  VariantControl=Phasor
  vqd+- : Outport
  iqd+- : Outport  Port=2
  freq : Outport  Port=3
  theta : Outport  Port=4
  PQabc : Outport  Port=5

== system Scenario_3_v2/G1/VSC v2/VSC Control/Modulation ==
  note: 1) Add Subsystem or Model blocks as valid variant choices.
      | 2) You cannot connect blocks at this level. At simulation, connectivity is automatically
      | determined, based on the active variant and port name matching.
  vqd+- : Inport
  vqd+-* : Inport  Port=2
  iqd+-* : Inport  Port=3
  theta : Inport  Port=4
  EMT AVG : Subsystem  VariantControl=EMT_AVG
  EMT Switching : Subsystem  VariantControl=EMT_SW
  Phasor I and Phasor PQ : Subsystem  VariantControl=Phasor_I_and_PQ
  Phasor Quasi-EMT : Subsystem  VariantControl=Phasor_QEMT
  Ref : Outport

== system Scenario_3_v2/G1/VSC v2/VSC Model/EMT AVG ==
  Ref : Inport
  Controlled Voltage Source3 : powerlib/Electrical Sources/Controlled Voltage Source  Initialize=off  Source_Type=AC  Amplitude=abs(Vc)*sqrt(2)  Phase=angle(Vc)  Frequency=fg  Measurements=None
  Controlled Voltage Source4 : powerlib/Electrical Sources/Controlled Voltage Source  Initialize=off  Source_Type=AC  Amplitude=abs(Vc)*sqrt(2)  Phase=angle(Vc)-2*pi/3  Frequency=fg  Measurements=None
  Controlled Voltage Source5 : powerlib/Electrical Sources/Controlled Voltage Source  Initialize=off  Source_Type=AC  Amplitude=abs(Vc)*sqrt(2)  Phase=angle(Vc)+2*pi/3  Frequency=fg  Measurements=None
  Demux1 : Demux  Outputs=3
  Ground : powerlib/Elements/Ground  LConnTagsString=a
  Ground4 : powerlib/Elements/Ground  LConnTagsString=a
  Ground5 : powerlib/Elements/Ground  LConnTagsString=a
  Ini Vabc : Subsystem
  A : PMIOPort  Side=Left
  B : PMIOPort  Port=2  Side=Left
  C : PMIOPort  Port=3  Side=Left
  wires:
  Demux1/1 -> Controlled Voltage Source3/1
  Demux1/2 -> Controlled Voltage Source4/1
  Demux1/3 -> Controlled Voltage Source5/1
  Ref/1 -> Ini Vabc/1(Vabc)
  Ini Vabc/1(out) -> Demux1/1
  connections:
  Ground/LConn1 -- Controlled Voltage Source3/LConn1
  Ground4/LConn1 -- Controlled Voltage Source4/LConn1
  Ground5/LConn1 -- Controlled Voltage Source5/LConn1
  Controlled Voltage Source3/RConn1 -- A/RConn1
  Controlled Voltage Source4/RConn1 -- B/RConn1
  Controlled Voltage Source5/RConn1 -- C/RConn1

== system Scenario_3_v2/G1/VSC v2/VSC Model/EMT SW ==
  Ref : Inport
  DC Voltage Source : powerlib/Electrical Sources/DC Voltage Source  Amplitude=Vdc  Measurements=None
  Universal Bridge : powerlib/Power Electronics/Universal Bridge  Arms=3  SnubberResistance=1e6  SnubberCapacitance=inf  Device=IGBT / Diodes  Ron=1e-4  Lon=0  ForwardVoltages="[  0  0  ]"  ForwardVoltage=0  GTOparameters=[ 10e-6 , 20e-6 ]  IGBTparameters=[ 1e-6 , 2e-6 ]  Measurements=None  Measurements_2=None  converterType=Rectifier
  A : PMIOPort  Side=Left
  B : PMIOPort  Port=2  Side=Left
  C : PMIOPort  Port=3  Side=Left
  wires:
  Ref/1 -> Universal Bridge/1
  connections:
  Universal Bridge/LConn2 -- B/RConn1
  Universal Bridge/LConn1 -- A/RConn1
  Universal Bridge/LConn3 -- C/RConn1
  Universal Bridge/RConn1 -- DC Voltage Source/RConn1
  Universal Bridge/RConn2 -- DC Voltage Source/LConn1

== system Scenario_3_v2/G1/VSC v2/VSC Model/Phasor ==
  Ref : Inport
  Controlled Current Source : powerlib/Electrical Sources/Controlled Current Source  Initialize=off  Source_Type=AC  Amplitude=0  Phase=0  Frequency=0  Measurements=None
  Controlled Current Source1 : powerlib/Electrical Sources/Controlled Current Source  Initialize=off  Source_Type=AC  Amplitude=0  Phase=0  Frequency=0  Measurements=None
  Controlled Current Source2 : powerlib/Electrical Sources/Controlled Current Source  Initialize=off  Source_Type=AC  Amplitude=0  Phase=0  Frequency=0  Measurements=None
  Demux1 : Demux  Outputs=3
  Ground{1..3,5} (4 alike) : powerlib/Elements/Ground  LConnTagsString=a
  Three-Phase Series RLC Branch : powerlib/Elements/Three-Phase Series RLC Branch  LConnTagsString=A|B|C  RConnTagsString=A|B|C  BranchType=R  Resistance=1e7  Inductance=1e-3  Capacitance=1e-6  Measurements=None
  A : PMIOPort  Side=Left
  B : PMIOPort  Port=2  Side=Left
  C : PMIOPort  Port=3  Side=Left
  wires:
  Demux1/3 -> [c]
  Demux1/2 -> [b]
  Demux1/1 -> [a]
  Ref/1 -> Demux1/1
  [a] -> Controlled Current Source/1
  [b] -> Controlled Current Source1/1
  [c] -> Controlled Current Source2/1
  connections:
  Three-Phase Series RLC Branch/LConn1 -- Controlled Current Source/RConn1 -- A/RConn1
  Three-Phase Series RLC Branch/LConn3 -- Controlled Current Source2/RConn1 -- C/RConn1
  Ground5/LConn1 -- Three-Phase Series RLC Branch/RConn2 -- Three-Phase Series RLC Branch/RConn1 -- Three-Phase Series RLC Branch/RConn3
  Three-Phase Series RLC Branch/LConn2 -- Controlled Current Source1/RConn1 -- B/RConn1
  Controlled Current Source/LConn1 -- Ground1/LConn1
  Ground2/LConn1 -- Controlled Current Source1/LConn1
  Ground3/LConn1 -- Controlled Current Source2/LConn1

== system Scenario_3_v2/G10/VSC v2/VSC Control/Control loops ==
  note: 1) Add Subsystem or Model blocks as valid variant choices.
      | 2) You cannot connect blocks at this level. At simulation, connectivity is automatically
      | determined, based on the active variant and port name matching.
  Pset : Inport
  Qset : Inport  Port=2
  vqd+- : Inport  Port=3
  iqd+- : Inport  Port=4
  freq : Inport  Port=5
  Block : Inport  Port=6
  Edc : Inport  Port=7
  Phasor I 1st : Subsystem  VariantControl=Phasor_I_1st
  Phasor I ref : Subsystem  VariantControl=Phasor_I_ref
  Phasor PQ 1st : Subsystem  VariantControl=Phasor_PQ
  "SW, EMT AVG, Phasor Quasi-EMT" : Subsystem  VariantControl=EMT_and_QEMT
  vqd+-ref : Outport
  iqd+-ref : Outport  Port=2
  m : Outport  Port=3

== system Scenario_3_v2/G10/VSC v2/VSC Control/Measurements ==
  note: 1) Add Subsystem or Model blocks as valid variant choices.
      | 2) You cannot connect blocks at this level. At simulation, connectivity is automatically
      | determined, based on the active variant and port name matching.
  Vabc : Inport
  Iabc : Inport  Port=2
  EMT : Subsystem  VariantControl=EMT
  Phasor : Subsystem  VariantControl=Phasor
  vqd+- : Outport
  iqd+- : Outport  Port=2
  freq : Outport  Port=3
  theta : Outport  Port=4
  PQabc : Outport  Port=5

== system Scenario_3_v2/G10/VSC v2/VSC Control/Modulation ==
  note: 1) Add Subsystem or Model blocks as valid variant choices.
      | 2) You cannot connect blocks at this level. At simulation, connectivity is automatically
      | determined, based on the active variant and port name matching.
  vqd+- : Inport
  vqd+-* : Inport  Port=2
  iqd+-* : Inport  Port=3
  theta : Inport  Port=4
  EMT AVG : Subsystem  VariantControl=EMT_AVG
  EMT Switching : Subsystem  VariantControl=EMT_SW
  Phasor I and Phasor PQ : Subsystem  VariantControl=Phasor_I_and_PQ
  Phasor Quasi-EMT : Subsystem  VariantControl=Phasor_QEMT
  Ref : Outport

== system Scenario_3_v2/G10/VSC v2/VSC Model/EMT AVG ==
  Ref : Inport
  Controlled Voltage Source3 : powerlib/Electrical Sources/Controlled Voltage Source  Initialize=off  Source_Type=AC  Amplitude=abs(Vc)*sqrt(2)  Phase=angle(Vc)  Frequency=fg  Measurements=None
  Controlled Voltage Source4 : powerlib/Electrical Sources/Controlled Voltage Source  Initialize=off  Source_Type=AC  Amplitude=abs(Vc)*sqrt(2)  Phase=angle(Vc)-2*pi/3  Frequency=fg  Measurements=None
  Controlled Voltage Source5 : powerlib/Electrical Sources/Controlled Voltage Source  Initialize=off  Source_Type=AC  Amplitude=abs(Vc)*sqrt(2)  Phase=angle(Vc)+2*pi/3  Frequency=fg  Measurements=None
  Demux1 : Demux  Outputs=3
  Ground : powerlib/Elements/Ground  LConnTagsString=a
  Ground4 : powerlib/Elements/Ground  LConnTagsString=a
  Ground5 : powerlib/Elements/Ground  LConnTagsString=a
  A : PMIOPort  Side=Left
  B : PMIOPort  Port=2  Side=Left
  C : PMIOPort  Port=3  Side=Left
  wires:
  Ref/1 -> Demux1/1
  Demux1/1 -> Controlled Voltage Source3/1
  Demux1/2 -> Controlled Voltage Source4/1
  Demux1/3 -> Controlled Voltage Source5/1
  connections:
  Ground/LConn1 -- Controlled Voltage Source3/LConn1
  Ground4/LConn1 -- Controlled Voltage Source4/LConn1
  Ground5/LConn1 -- Controlled Voltage Source5/LConn1
  Controlled Voltage Source3/RConn1 -- A/RConn1
  Controlled Voltage Source4/RConn1 -- B/RConn1
  Controlled Voltage Source5/RConn1 -- C/RConn1

== system Scenario_3_v2/G10/VSC v2/VSC Model/EMT SW ==
  Ref : Inport
  DC Voltage Source : powerlib/Electrical Sources/DC Voltage Source  Amplitude=Vdc  Measurements=None
  Universal Bridge : powerlib/Power Electronics/Universal Bridge  Arms=3  SnubberResistance=1e6  SnubberCapacitance=inf  Device=IGBT / Diodes  Ron=1e-4  Lon=0  ForwardVoltages="[  0  0  ]"  ForwardVoltage=0  GTOparameters=[ 10e-6 , 20e-6 ]  IGBTparameters=[ 1e-6 , 2e-6 ]  Measurements=None  Measurements_2=None  converterType=Rectifier
  A : PMIOPort  Side=Left
  B : PMIOPort  Port=2  Side=Left
  C : PMIOPort  Port=3  Side=Left
  wires:
  Ref/1 -> Universal Bridge/1
  connections:
  Universal Bridge/LConn2 -- B/RConn1
  Universal Bridge/LConn1 -- A/RConn1
  Universal Bridge/LConn3 -- C/RConn1
  Universal Bridge/RConn1 -- DC Voltage Source/RConn1
  Universal Bridge/RConn2 -- DC Voltage Source/LConn1

== system Scenario_3_v2/G10/VSC v2/VSC Model/Phasor ==
  Ref : Inport
  Controlled Current Source : powerlib/Electrical Sources/Controlled Current Source  Initialize=off  Source_Type=AC  Amplitude=0  Phase=0  Frequency=0  Measurements=None
  Controlled Current Source1 : powerlib/Electrical Sources/Controlled Current Source  Initialize=off  Source_Type=AC  Amplitude=0  Phase=0  Frequency=0  Measurements=None
  Controlled Current Source2 : powerlib/Electrical Sources/Controlled Current Source  Initialize=off  Source_Type=AC  Amplitude=0  Phase=0  Frequency=0  Measurements=None
  Demux1 : Demux  Outputs=3
  Ground{1..3,5} (4 alike) : powerlib/Elements/Ground  LConnTagsString=a
  Three-Phase Series RLC Branch : powerlib/Elements/Three-Phase Series RLC Branch  LConnTagsString=A|B|C  RConnTagsString=A|B|C  BranchType=R  Resistance=1e7  Inductance=1e-3  Capacitance=1e-6  Measurements=None
  A : PMIOPort  Side=Left
  B : PMIOPort  Port=2  Side=Left
  C : PMIOPort  Port=3  Side=Left
  wires:
  Demux1/3 -> [c]
  Demux1/2 -> [b]
  Demux1/1 -> [a]
  Ref/1 -> Demux1/1
  [a] -> Controlled Current Source/1
  [b] -> Controlled Current Source1/1
  [c] -> Controlled Current Source2/1
  connections:
  Three-Phase Series RLC Branch/LConn1 -- Controlled Current Source/RConn1 -- A/RConn1
  Three-Phase Series RLC Branch/LConn3 -- Controlled Current Source2/RConn1 -- C/RConn1
  Ground5/LConn1 -- Three-Phase Series RLC Branch/RConn2 -- Three-Phase Series RLC Branch/RConn1 -- Three-Phase Series RLC Branch/RConn3
  Three-Phase Series RLC Branch/LConn2 -- Controlled Current Source1/RConn1 -- B/RConn1
  Controlled Current Source/LConn1 -- Ground1/LConn1
  Ground2/LConn1 -- Controlled Current Source1/LConn1
  Ground3/LConn1 -- Controlled Current Source2/LConn1

== system Scenario_3_v2/G12/VSC v2/VSC Control/Control loops ==
  note: 1) Add Subsystem or Model blocks as valid variant choices.
      | 2) You cannot connect blocks at this level. At simulation, connectivity is automatically
      | determined, based on the active variant and port name matching.
  Pset : Inport
  Qset : Inport  Port=2
  vqd+- : Inport  Port=3
  iqd+- : Inport  Port=4
  freq : Inport  Port=5
  Block : Inport  Port=6
  Edc : Inport  Port=7
  Phasor I 1st : Subsystem  VariantControl=Phasor_I_1st
  Phasor I ref : Subsystem  VariantControl=Phasor_I_ref
  Phasor PQ 1st : Subsystem  VariantControl=Phasor_PQ
  "SW, EMT AVG, Phasor Quasi-EMT" : Subsystem  VariantControl=EMT_and_QEMT
  vqd+-ref : Outport
  iqd+-ref : Outport  Port=2
  m : Outport  Port=3

== system Scenario_3_v2/G12/VSC v2/VSC Control/Measurements ==
  note: 1) Add Subsystem or Model blocks as valid variant choices.
      | 2) You cannot connect blocks at this level. At simulation, connectivity is automatically
      | determined, based on the active variant and port name matching.
  Vabc : Inport
  Iabc : Inport  Port=2
  EMT : Subsystem  VariantControl=EMT
  Phasor : Subsystem  VariantControl=Phasor
  vqd+- : Outport
  iqd+- : Outport  Port=2
  freq : Outport  Port=3
  theta : Outport  Port=4
  PQabc : Outport  Port=5

== system Scenario_3_v2/G12/VSC v2/VSC Control/Modulation ==
  note: 1) Add Subsystem or Model blocks as valid variant choices.
      | 2) You cannot connect blocks at this level. At simulation, connectivity is automatically
      | determined, based on the active variant and port name matching.
  vqd+- : Inport
  vqd+-* : Inport  Port=2
  iqd+-* : Inport  Port=3
  theta : Inport  Port=4
  EMT AVG : Subsystem  VariantControl=EMT_AVG
  EMT Switching : Subsystem  VariantControl=EMT_SW
  Phasor I and Phasor PQ : Subsystem  VariantControl=Phasor_I_and_PQ
  Phasor Quasi-EMT : Subsystem  VariantControl=Phasor_QEMT
  Ref : Outport

== system Scenario_3_v2/G12/VSC v2/VSC Model/EMT AVG ==
  Ref : Inport
  Controlled Voltage Source3 : powerlib/Electrical Sources/Controlled Voltage Source  Initialize=off  Source_Type=AC  Amplitude=abs(Vc)*sqrt(2)  Phase=angle(Vc)  Frequency=fg  Measurements=None
  Controlled Voltage Source4 : powerlib/Electrical Sources/Controlled Voltage Source  Initialize=off  Source_Type=AC  Amplitude=abs(Vc)*sqrt(2)  Phase=angle(Vc)-2*pi/3  Frequency=fg  Measurements=None
  Controlled Voltage Source5 : powerlib/Electrical Sources/Controlled Voltage Source  Initialize=off  Source_Type=AC  Amplitude=abs(Vc)*sqrt(2)  Phase=angle(Vc)+2*pi/3  Frequency=fg  Measurements=None
  Demux1 : Demux  Outputs=3
  Ground : powerlib/Elements/Ground  LConnTagsString=a
  Ground4 : powerlib/Elements/Ground  LConnTagsString=a
  Ground5 : powerlib/Elements/Ground  LConnTagsString=a
  A : PMIOPort  Side=Left
  B : PMIOPort  Port=2  Side=Left
  C : PMIOPort  Port=3  Side=Left
  wires:
  Ref/1 -> Demux1/1
  Demux1/1 -> Controlled Voltage Source3/1
  Demux1/2 -> Controlled Voltage Source4/1
  Demux1/3 -> Controlled Voltage Source5/1
  connections:
  Ground/LConn1 -- Controlled Voltage Source3/LConn1
  Ground4/LConn1 -- Controlled Voltage Source4/LConn1
  Ground5/LConn1 -- Controlled Voltage Source5/LConn1
  Controlled Voltage Source3/RConn1 -- A/RConn1
  Controlled Voltage Source4/RConn1 -- B/RConn1
  Controlled Voltage Source5/RConn1 -- C/RConn1

== system Scenario_3_v2/G12/VSC v2/VSC Model/EMT SW ==
  Ref : Inport
  DC Voltage Source : powerlib/Electrical Sources/DC Voltage Source  Amplitude=Vdc  Measurements=None
  Universal Bridge : powerlib/Power Electronics/Universal Bridge  Arms=3  SnubberResistance=1e6  SnubberCapacitance=inf  Device=IGBT / Diodes  Ron=1e-4  Lon=0  ForwardVoltages="[  0  0  ]"  ForwardVoltage=0  GTOparameters=[ 10e-6 , 20e-6 ]  IGBTparameters=[ 1e-6 , 2e-6 ]  Measurements=None  Measurements_2=None  converterType=Rectifier
  A : PMIOPort  Side=Left
  B : PMIOPort  Port=2  Side=Left
  C : PMIOPort  Port=3  Side=Left
  wires:
  Ref/1 -> Universal Bridge/1
  connections:
  Universal Bridge/LConn2 -- B/RConn1
  Universal Bridge/LConn1 -- A/RConn1
  Universal Bridge/LConn3 -- C/RConn1
  Universal Bridge/RConn1 -- DC Voltage Source/RConn1
  Universal Bridge/RConn2 -- DC Voltage Source/LConn1
